simulink model "Experiment_0310yice_cs"  (R2019a)
settings: Solver=ode5  StartTime=0.0  StopTime=20  FixedStep=1/100  RelTol=1e-3
PreLoadFcn:
  | mbxruntime.callbacks.PreLoadFcn(bdroot);
PostLoadFcn:
  | mbxruntime.callbacks.PostLoadFcn(bdroot);
InitFcn:
  | mbxruntime.callbacks.InitFcn(bdroot);
StartFcn:
  | mbxruntime.callbacks.StartFcn(bdroot);
StopFcn:
  | mbxruntime.callbacks.StopFcn(bdroot);
model workspace (MAT data in the model file):
  mbox_table : struct (value not decoded)
  model_closed = 0
  sim_status = 0
undefined symbols (not defined in the file or in its folder): DiscIntNeverNeededParam, InitImageOutputDir
libraries: PreScanSimulinkLibrary x20, simulink_extras x1
(part 1 of 2)
CloseFcn:
  | mbxruntime.callbacks.CloseFcn(bdroot);
settings Model: NumberOfSteps=10  Creator=PRESCAN  LastModifiedBy=HP
settings DataIOCC: LimitDataPoints=on  SaveFormat=Array  SignalLoggingSaveFormat=ModelDataLogs  ReturnWorkspaceOutputs=off
settings OptimizationCC: ExpressionDepthLimit=2147483647  InitFltsAndDblsToZero=on  LifeSpan=inf
settings DebuggingCC: SaveWithParameterizedLinksMsg=none  UnderspecifiedInitializationDetection=Classic  MergeDetectMultiDrivingBlocksExec=none  SignalResolutionControl=TryResolveAllWithWarning  MultiTaskDSMMsg=warning  MultiTaskCondExecSysMsg=none  FcnCallInpInsideContextMsg=warning  StateNameClashWarn=warning  SFUnexpectedBacktrackingDiag=warning  SFNoUnconditionalDefaultTransitionDiag=warning  SFExecutionAtInitializationDiag=none  ArithmeticOperatorsInVariantConditions=warning
settings HardwareCC: ProdBitPerPointer=32  ProdBitPerSizeT=32  ProdBitPerPtrDiffT=32  ProdLargestAtomicFloat=None  ProdIntDivRoundTo=Undefined  ProdEndianess=Unspecified  ProdWordSize=32  ProdHWDeviceType=32-bit Generic
settings ModelReferenceCC: UpdateModelReferenceTargets=IfOutOfDate  PropagateSignalLabelsOutOfModel=off
settings SFSimCC: SimUseLocalCustomCode=off  SimParseCustomCode=off
settings SFSimCC: SimCustomHeaderCode=|
  | #include "prescan.h"
  | #include "prescan_platform.h"
settings RTWCC: RTWUseLocalCustomCode=off
settings CodeAppCC: StateflowObjectComments=on
settings GRTTargetCC: TargetFcnLib=ansi_tfl_tmw.mat  TargetLangStandard=C89/C90 (ANSI)  GeneratePreprocessorConditionals=Disable all  CombineOutputUpdateFcns=off  GRTInterface=on
settings ConfigComp: CovMetricSettings=dw  CovHtmlReporting=on  CovSaveCumulativeToWorkspaceVar=on  CovSaveSingleToWorkspaceVar=on  CovExternalEMLEnable=off

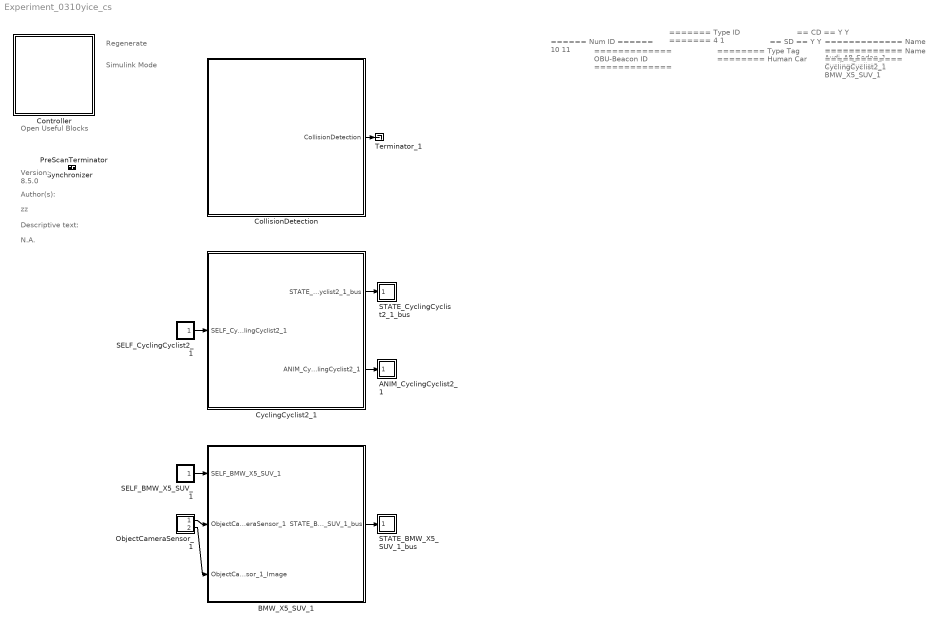
== system Experiment_0310yice_cs ==
  note: Regenerate
  note: Simulink Mode
  note: Open Useful Blocks
  note: 8.5.0
  note: Version:
  note: Author(s):
  note: zz
  note: Descriptive text:
  note: N.A.
  note: =============
      | Name
      | =============
      | Audi_A8_Sedan_1
      | CyclingCyclist2_1
  note: ======
      | Num ID
      | ======
      | 10
      | 11
  note: =============
      | OBU-Beacon ID
      | =============
  note: =======
      | Type ID
      | =======
      | 4
      | 1
  note: ========
      | Type Tag
      | ========
      | Human
      | Car
  note: ==
      | SD
      | ==
      | Y
      | Y
  note: ==
      | CD
      | ==
      | Y
      | Y
  note: =============
      | Name
      | =============
      | CyclingCyclist2_1
      | BMW_X5_SUV_1
  ANIM_CyclingCyclist2_1 : Subsystem  Tag=actuator/AnimationOutport  Priority=0  LoadFcn=load('PreScanAnimActuatorData.mat')  mask(PreScan Sink Block: State Animation){}
      mask help: The Cyclist Animation port allows the cyclist to ride the bicycle.
      settings: OpenFcn=open_system([gcb '/Actuator'],'mask')
      mask Help: eval('openHelp(239)')
      mask Display: image(imread('CyclingCyclist2.jpg'))
  BMW_X5_SUV_1 : Subsystem  Tag=WorldObjectSubSystem  InitFcn=UniqueId = '197';
      mask init:
      | modelPath = GenericModelHelper.getGenericModelFilePath('ModelDepo','Vehicles\BMW_X5\BMW_X5.pgmb','cea918691563e9ae3e6a88ec95e6726a');imagePath = GenericModelHelper.getCompilationPicture(modelPath, 'BMW_X5_HighPoly.png');
      mask Display: image(imread(imagePath));color('white');text(0, 0, ' ID=11\n')
  CollisionDetection : Subsystem  Tag=sensor/CollisionDetection  Priority=3  LoadFcn=load('PrescanCollisionDetectionData.mat');load('PrescanCollisionDetectionMessage.mat')  mask(PreScan Source Block: CollisionDetection){}
      mask help: Collision Detection can be used to detect collisions between PreScan components. For Collision Detection the actual component shape is taken into account, so it is not a bounding box approach.
      settings: OpenFcn=open_system([gcb '/Sensor'],'mask')
      mask Help: eval('openHelp(811)')
      mask Display: image(imread('crash.jpg'))
  Controller : Subsystem  Description=C9959BB6F9C6CCCA2A6EA89AF77C45A9E7A5C62A073B3FDCE97DBD876D9D5A7D  Priority=-1  LoadFcn=load PreScanControllerData  mask(PreScan Simulation Controller){prescanversion='8.5.0', ModelReferencing=off, TimeStep=5/100, ControlMode=0, PreScanExecutionMode=on, ControllerCount=0, ControllerIndex=0, ControllerOptions=''}
      mask prompts: prescanversion "PreScan Version"; ModelReferencing "Use Model Referencing"; TimeStep "Upload Period [s]"; ControlMode "Control Mode"; PreScanExecutionMode "Execution Mode"; ControllerCount "Controller Count"; ControllerIndex "Controller Index"; ControllerOptions "Controller Options"
      mask help:
      | Please do not remove this block from the compilation sheet,
      | as it connects the model to the PreScan environment.
      mask init:
      | model = bdroot(gcb);
      | ExperimentFile = mbxruntime.findExperimentFile(model,true); %relative path
      | 
      | [d1, d2, d3, prescandata] = prescan_Settings();
      | ModelDepo = fullfile(prescandata,'ModelDepo'); 
      | 
      | RTmode = mbxruntime.getRTMode(model);
      | 
      | SimulationMode = get_param(bdroot,'SimulationMode');
      | if strcmp(SimulationMode, 'rapid-accelerator')
      |     SimulationMode = 'external';
      | end
      | TargetName = get_param(bdroot,'SystemTargetFile');
      settings: ModelCloseFcn=assignin('base',['model_closed_' bdroot],true);
      mask Help: eval('openHelp(812)')
      mask Display: image(imread('prescanlogo.ico'))
  CyclingCyclist2_1 : Subsystem  Tag=WorldObjectSubSystem  InitFcn=UniqueId = '71';
      mask init:
      | imagePath=which('CyclingCyclist2.jpg');
      mask Display: image(imread(imagePath));color('white');text(0, 0, ' ID=10\n')
  ObjectCameraSensor_1 : Subsystem  Tag=sensor/ObjectCamera/data  Priority=3  LoadFcn=load('PrescanOCSData.mat');load('PrescanOCSMessage.mat')  mask(PreScan Source Block: Object Camera Sensor){}
      mask help: The Object Camera Sensor provides information on objects locations.
      settings: OpenFcn=open_system([gcb '/Sensor'],'mask')
      mask Help: eval('openHelp(2401)')
      mask Display: image(imread('ObjectCameraSensorSL.png'))
  PreScanTerminator : Subsystem  Tag=PreScanTerminator  Priority=999  LoadFcn=load PrescanTerminatorData  mask(PreScan Simulation Terminator){TimeStep=5/100}
      mask prompts: TimeStep "Upload Period [s]"
      mask help:
      | Please do not remove this block from the compilation sheet as it
      | connects the model to the PreScan environment.
      mask Help: eval('openHelp(812)')
      mask Display: image(imread('prescanlogo.ico'))
  SELF_BMW_X5_SUV_1 : Subsystem  Tag=sensor/SelfPort  Priority=3  LoadFcn=load('PreScanSelfSensorData.mat')  mask(PreScan Source Block: SELF){}
      mask help:
      | The SELF port shows (state) information of the actor itself. The outputs are position in the experiment's axis system and the GPS coordinates, and the object's absolute velocity and compass heading.
      |
      | For more information, please click Help.
      settings: OpenFcn=open_system([gcb '/Sensor'],'mask')
      mask Help: eval('openHelp(462)')
      mask Display: image(imread('GPS.png'))
  SELF_CyclingCyclist2_1 : Subsystem  Tag=sensor/SelfPort  Priority=3  LoadFcn=load('PreScanSelfSensorData.mat')  mask(PreScan Source Block: SELF){}
      mask help:
      | The SELF port shows (state) information of the actor itself. The outputs are position in the experiment's axis system and the GPS coordinates, and the object's absolute velocity and compass heading.
      |
      | For more information, please click Help.
      settings: OpenFcn=open_system([gcb '/Sensor'],'mask')
      mask Help: eval('openHelp(462)')
      mask Display: image(imread('GPS.png'))
  STATE_BMW_X5_SUV_1_bus : Subsystem  Tag=actuator/StatePort  Priority=0  LoadFcn=load('PreScanStateActuatorData.mat')  mask(PreScan Sink Block: State){}
      mask help:
      | The Actor State contains a vector signal of size (9x1), containing the following signals:
      |
      | -  Position    	(x,y,z)             	[m]
      | -  Velocity    	(vx,vy,vz)         	[m/s]
      | -  Angles       	(Roll, Pitch, Yaw)	[rad]
      |
      | The Actor state is defined in the global axis system.
      | The state is superponed on the Initial position defined in the GUI.
      |
      | For more information, please click Help.
      settings: OpenFcn=open_system([gcb '/Actuator'],'mask')
      mask Help: eval('openHelp(222)')
      mask Display: image(imread('State.png'))
  STATE_CyclingCyclist2_1_bus : Subsystem  Tag=actuator/StatePort  Priority=0  LoadFcn=load('PreScanStateActuatorData.mat')  mask(PreScan Sink Block: State){}
      mask help:
      | The Actor State contains a vector signal of size (9x1), containing the following signals:
      |
      | -  Position    	(x,y,z)             	[m]
      | -  Velocity    	(vx,vy,vz)         	[m/s]
      | -  Angles       	(Roll, Pitch, Yaw)	[rad]
      |
      | The Actor state is defined in the global axis system.
      | The state is superponed on the Initial position defined in the GUI.
      |
      | For more information, please click Help.
      settings: OpenFcn=open_system([gcb '/Actuator'],'mask')
      mask Help: eval('openHelp(222)')
      mask Display: image(imread('State.png'))
  Synchronizer : Subsystem  Tag=PreScanSynchronizer  Priority=1  LoadFcn=load PrescanSynchronizeData  mask(PreScan Simulation Core Block){TimeStep=5/100}
      mask prompts: TimeStep "Timestep [s]"
      mask help:
      | Please do not remove this block from the PreScan compilation sheet,
      | as it contains essential configuration parameters for a PreScan simulation.
      settings: DeleteFcn=PreScanBlockDeleteFcn;
      mask Display: image(imread('prescanlogo.ico'))
  Terminator_1 : Terminator
  wires:
  CyclingCyclist2_1/1(STATE_CyclingCyclist2_1_bus) -> STATE_CyclingCyclist2_1_bus/1(STATE_CyclingCyclist2_1_bus)
  CyclingCyclist2_1/2(ANIM_CyclingCyclist2_1) -> ANIM_CyclingCyclist2_1/1(ANIM_CyclingCyclist2_1)
  SELF_CyclingCyclist2_1/1(SELF_CyclingCyclist2_1) -> CyclingCyclist2_1/1(SELF_CyclingCyclist2_1)
  CollisionDetection/1(CollisionDetection) -> Terminator_1/1
  BMW_X5_SUV_1/1(STATE_BMW_X5_SUV_1_bus) -> STATE_BMW_X5_SUV_1_bus/1(STATE_BMW_X5_SUV_1_bus)
  SELF_BMW_X5_SUV_1/1(SELF_BMW_X5_SUV_1) -> BMW_X5_SUV_1/1(SELF_BMW_X5_SUV_1)
  ObjectCameraSensor_1/1(ObjectCameraSensor_1) -> BMW_X5_SUV_1/2(ObjectCameraSensor_1)
  ObjectCameraSensor_1/2(ObjectCameraSensor_1_Image) -> BMW_X5_SUV_1/3(ObjectCameraSensor_1_Image)

== system Experiment_0310yice_cs/ANIM_CyclingCyclist2_1 ==
  ANIM_CyclingCyclist2_1 : Inport  Tag=inport/AnimationOutport  OutDataTypeStr=Bus: PRESCAN_ANIMACTUATORDATA  PortDimensions=2  SampleTime=5/100  BusOutputAsStruct=on
  Actuator : S-Function  FunctionName=sfun_CyclistAnimActuator  Parameters=UniqueID, uint8([ParentObject 0]), TimeStep  SFunctionDeploymentMode=off  EnableBusSupport=off  mask(PreScan Sink Block: State Animation){UniqueID=71, ParentObject=CyclingCyclist2_1, TimeStep=5/100}
      mask prompts: UniqueID "Auto-Assigned: Unique ID"; ParentObject "Auto-Assigned: ParentObject"; TimeStep "Auto-Assigned: Upload Period [s]"
      mask help: The Cyclist Animation port allows the cyclist to ride the bicycle.
      mask Help: eval('openHelp(239)')
      mask Display: image(imread('CyclingCyclist2.jpg'))
  wires:
  ANIM_CyclingCyclist2_1/1 -> Actuator/1

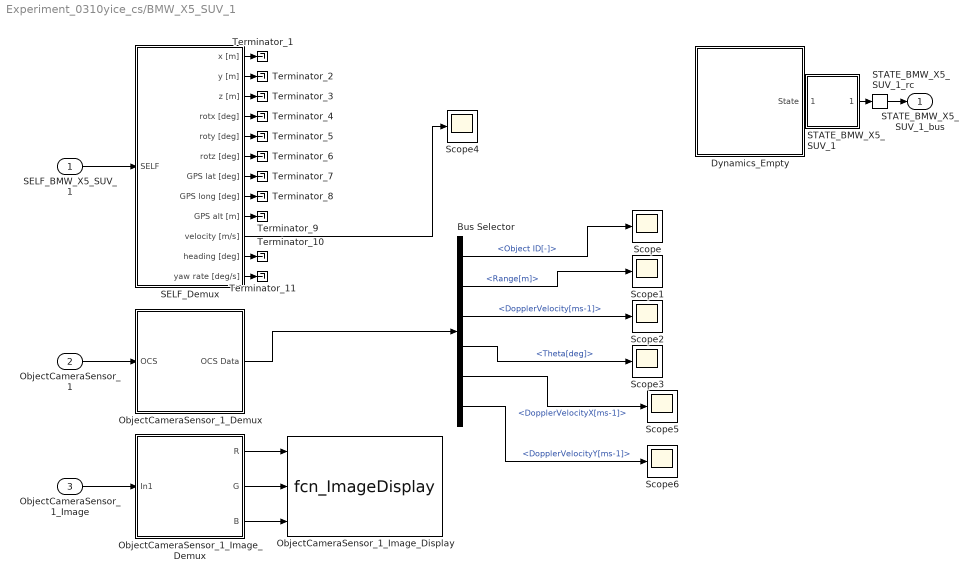
== system Experiment_0310yice_cs/BMW_X5_SUV_1 ==
  SELF_BMW_X5_SUV_1 : Inport  Tag=inport/SelfPort  OutDataTypeStr=Bus: PRESCAN_SELFSENSORDATA  PortDimensions=1  SampleTime=5/100  BusOutputAsStruct=on
  ObjectCameraSensor_1 : Inport  Tag=inport/ObjectCamera/data  Port=2  OutDataTypeStr=Bus: PRESCAN_OCS_MESSAGE  PortDimensions=3  SampleTime=1/20  BusOutputAsStruct=on
  ObjectCameraSensor_1_Image : Inport  Tag=inport/ObjectCamera/image  Port=3  OutDataTypeStr=uint8  SampleTime=1/20  BusOutputAsStruct=on
  Bus Selector : BusSelector  OutputSignals=Object ID[-],Range[m],DopplerVelocity[ms-1],Theta[deg],DopplerVelocityX[ms-1],DopplerVelocityY[ms-1]
  Dynamics_Empty : Subsystem  Tag=Dynamics_Empty
      mask Help: eval('openHelp(202)')
      mask Display: port_label('output', 1, 'State');text(0,0,' Empty\n')
  ObjectCameraSensor_1_Demux : Subsystem  Tag=demux/OCS  mask(PreScan Demux Block: Object Camera Sensor){detectableObjects=3}
      mask prompts: detectableObjects "Max. detectable objects"
      settings: DeleteFcn=PreScanBlockDeleteFcn;
      mask Help: eval('openHelp(2401)')
      mask Display:
      | port_label('input', 1, 'OCS')
      | port_label('output', 1, 'OCS Data')
  ObjectCameraSensor_1_Image_Demux : Subsystem  Tag=demux/Camera/Color  mask{SensorName=ObjectCameraSensor_1, hres=320, vres=240}
      mask prompts: SensorName "Sensor Name"; hres "Horizontal Resolution"; vres "Vertical Resolution"
      mask Help: eval('openHelp(2401)')
      mask Display:
      | fprintf('MONO CAMERA:\n Color\n %s \n %d x %d px',SensorName,hres,vres)
      | port_label('output',1,'R')
      | port_label('output',2,'G')
      | port_label('output',3,'B')
  ObjectCameraSensor_1_Image_Display : M-S-Function  Tag=CameraSensor_Color_Display  InitFcn=InitImageOutputDir(gcb);  FunctionName=fcn_ImageDisplay  Parameters=SensorName EnableDisplay EnablePosition DisplayPosition FigureHandle SaveResults BitmapFormat TempOutputDir CameraType DataType  mask(PreScan Color Display Block){SensorName=ObjectCameraSensor_1_Image, EnableDisplay=on, EnablePosition=off, DisplayPosition=[10 10 320 240], FigureHandle=19701, SaveResults=off, Format=PNG, TempOutputDir=0, CameraType=Mono, DataType=uint8}
      mask prompts: SensorName "User Specified: Title of Display"; EnableDisplay "Active"; EnablePosition "Set Display window position"; DisplayPosition "Display window position [xpos ypos width height]"; FigureHandle "Unique Handle"; SaveResults "Save results"; TempOutputDir "OutputDir"; CameraType "Camera Type"; DataType "Image Data Type"
      mask help: This block displays the RGB output of a PreScan camera sensor.
      mask init:
      | if EnableDisplay
      |     EnableString='';
      |     EnableColor='gray';
      | else
      |     EnableString='INACTIVE';
      |     EnableColor='red';
      | end
      | switch Format
      |     case 1
      |         BitmapFormat = 'png';
      |     case 2
      |         BitmapFormat = 'bmp';
      |     case 3
      |         BitmapFormat = 'jpg';
      | end 
      | if CameraType==1
      |     CameraTypeName='MONO';
      |     PortNumber=0;
      | else
      |     CameraTypeName='STEREO';
      |     PortNumber=3;
      | end
      settings: CopyFcn=CopyFcnDisplay  DeleteFcn=PreScanBlockDeleteFcn;  ModelCloseFcn=fcn_ImageDisplay_ModelCloseFcn
      mask Help: eval('openHelp(2401)')
      mask Callback EnablePosition:
      | MV=get_param(gcb,'MaskVisibilities');
      | if strcmp(get_param(gcb,'EnablePosition'),'on')
      |     MV{4}='on';
      | else
      |     MV{4}='off';
      | end
      | set_param(gcb,'MaskVisibilities',MV);
      | clear MV;
      mask TypeOptions Format: PNG | BMP | JPG
      mask TypeOptions CameraType: Mono | Stereo
      mask TypeOptions DataType: uint8 | single
      mask Display:
      | color(EnableColor);
      | fprintf('%s\n DISPLAY:\n Color \n %s',EnableString,SensorName)
      | port_label('input',1,'R')
      | port_label('input',2,'G')
      | port_label('input',3,'B')
      | port_label('input',PortNumber+1,'R')
      | port_label('input',PortNumber+2,'G')
      | port_label('input',PortNumber+3,'B')
  SELF_Demux : Subsystem  Tag=demux/SelfPort  mask(PreScan Demux Block:){}
      mask help:
      | The SELF port shows (state) information of the actor itself. The outputs are position in the experiment's axis system and the GPS coordinates, and the object's absolute velocity and compass heading.
      |
      | For more information, please click Help.
      settings: DeleteFcn=PreScanBlockDeleteFcn;
      mask Help: eval('openHelp(462)')
      mask Display:
      | port_label('output',1,'x [m]')
      | port_label('output',2,'y [m]')
      | port_label('output',3,'z [m]','texmode','on')
      | port_label('output',4,'Rotx [deg]','texmode','on')
      | port_label('output',5,'Roty [deg]','texmode','on')
      | port_label('output',6,'Rotz [deg]','texmode','on')
      | port_label('output',7,'GPS lat [deg]','texmode','on')
      | port_label('output',8,'GPS long [deg]','texmode','on')
      | port_label('output',9,'GPS alt [m]','texmode','on')
      | port_label('output',10,'Velocity [m/s]')
      | port_label('output',11,'Heading [deg]')
      | port_label('output',12,'Yaw rate [deg/s]')
  STATE_BMW_X5_SUV_1 : Subsystem  Tag=mux/StatePort  Priority=0  LoadFcn=load PrescanStateActuatorData  mask(PreScan Sink Block: State){x0=44.6973, y0=48.6545, z0=0.69, Roll0=0, Pitch0=0, Yaw0=90, TimeStep=1/100}
      mask prompts: x0 "Ini x-position VEHICLE wrt GLOBAL axis system [m]"; y0 "Ini y-position VEHICLE wrt GLOBAL axis system [m]"; z0 "Ini z-position VEHICLE wrt GLOBAL axis system [m]"; Roll0 "Ini roll-angle BODY wrt VEHICLE axis system [deg]"; Pitch0 "Ini pitch-angle BODY wrt VEHICLE axis system [deg]"; Yaw0 "Ini yaw-angle VEHICLE wrt GLOBAL axis system [deg]"; TimeStep "Auto-Assigned: Upload Period [s]"
      mask help:
      | The Actor State contains a vector signal of size (9x1), containing the following signals:
      |
      | -  Position                  (x,y,z)                                     [m]
      | -  Velocity                  (vx,vy,vz)                               [m/s]
      | -  Angles                    (Roll, Pitch, Yaw)                   [rad]
      |
      | The Actor state is defined in the global axis system.
      | The state is superponed on the Initial position defined in the GUI.
      |
      | For more information, please click Help.
      settings: DeleteFcn=PreScanBlockDeleteFcn;
      mask Help: eval('openHelp(222)')
      mask Display: image(imread('State.png'))
  STATE_BMW_X5_SUV_1_rc : RateTransition  Tag=mux_rc/StatePort  OutPortSampleTimeOpt=Inherit
  Scope{,1..6} (7 alike) : Scope
  Terminator_{1..11} (11 alike) : Terminator
  STATE_BMW_X5_SUV_1_bus : Outport  Tag=outport/StatePort  OutDataTypeStr=Bus: PRESCAN_STATEACTUATORDATA  PortDimensions=1  SampleTime=5/100
  wires:
  ObjectCameraSensor_1_Demux/1(OCS Data) -> Bus Selector/1
  Bus Selector/1 -> Scope/1  "<Object ID[-]>"
  Bus Selector/2 -> Scope1/1  "<Range[m]>"
  Bus Selector/3 -> Scope2/1  "<DopplerVelocity[ms-1]>"
  Bus Selector/4 -> Scope3/1  "<Theta[deg]>"
  SELF_Demux/10(velocity [m/s]) -> Scope4/1
  Bus Selector/5 -> Scope5/1  "<DopplerVelocityX[ms-1]>"
  Bus Selector/6 -> Scope6/1  "<DopplerVelocityY[ms-1]>"
  STATE_BMW_X5_SUV_1_rc/1 -> STATE_BMW_X5_SUV_1_bus/1
  STATE_BMW_X5_SUV_1/1(StateBus) -> STATE_BMW_X5_SUV_1_rc/1
  SELF_BMW_X5_SUV_1/1 -> SELF_Demux/1(SELF)
  ObjectCameraSensor_1/1 -> ObjectCameraSensor_1_Demux/1(OCS)
  ObjectCameraSensor_1_Image/1 -> ObjectCameraSensor_1_Image_Demux/1(In1)
  ObjectCameraSensor_1_Image_Demux/1(R) -> ObjectCameraSensor_1_Image_Display/1
  ObjectCameraSensor_1_Image_Demux/2(G) -> ObjectCameraSensor_1_Image_Display/2
  ObjectCameraSensor_1_Image_Demux/3(B) -> ObjectCameraSensor_1_Image_Display/3
  Dynamics_Empty/1(State) -> STATE_BMW_X5_SUV_1/1(State)
  SELF_Demux/1(x [m]) -> Terminator_1/1
  SELF_Demux/2(y [m]) -> Terminator_2/1
  SELF_Demux/3(z [m]) -> Terminator_3/1
  SELF_Demux/4(rotx [deg]) -> Terminator_4/1
  SELF_Demux/5(roty [deg]) -> Terminator_5/1
  SELF_Demux/6(rotz [deg]) -> Terminator_6/1
  SELF_Demux/7(GPS lat [deg]) -> Terminator_7/1
  SELF_Demux/8(GPS long [deg]) -> Terminator_8/1
  SELF_Demux/9(GPS alt [m]) -> Terminator_9/1
  SELF_Demux/11(heading [deg]) -> Terminator_10/1
  SELF_Demux/12(yaw rate [deg/s]) -> Terminator_11/1

== system Experiment_0310yice_cs/CollisionDetection ==
  Sensor : S-Function  FunctionName=sfun_CollisionDetection  Parameters=detectableCollisions, timestep  SFunctionDeploymentMode=off  EnableBusSupport=off  mask(PreScan Source Block: CollisionDetection){detectableCollisions=5, timestep=5/100}
      mask prompts: detectableCollisions "Max detectable collisions:"; timestep "MATLAB timestep:"
      mask help: Collision Detection can be used to detect collisions between PreScan components. For Collision Detection the actual component shape is taken into account, so it is not a bounding box approach.
      mask Help: eval('openHelp(811)')
      mask Display: image(imread('crash.jpg'))
  CollisionDetection : Outport  Tag=outport/CollisionDetection  OutDataTypeStr=Bus: PRESCAN_COLLISIONDETECTION_MESSAGE  PortDimensions=5  SampleTime=5/100
  wires:
  Sensor/1 -> CollisionDetection/1

== system Experiment_0310yice_cs/Controller ==
  Terminator : Terminator
  sfun_Controller : S-Function  FunctionName=sfun_Controller  Parameters=SParameter1, SParameter2, SParameter3, SParameter4, SParameter5, SParameter6, SParameter7, SParameter8, SParameter9, SParameter10, SampleTime  SFunctionDeploymentMode=off  EnableBusSupport=off  mask(Legacy Function){SFunctionSpec=void prescan_outputFcn(void** work1, PRESCAN_CONTROLLERDATA y1[1]), SParameter1=uint8([ExperimentFile 0]), SParameter2=uint8([ModelDepo 0]), SParameter3=uint8([ControllerOptions 0]), SParameter4=RTmode, SParameter5=PreScanExecutionMode, SParameter6=ControlMode, SParameter7=ControllerCount, SParameter8=ControllerIndex, SParameter9=uint8([SimulationMode 0]), SParameter10=uint8([TargetName 0]), SampleTime=TimeStep, ShowSpec=on}
      mask prompts: SParameter1 "P1:"; SParameter2 "P2:"; SParameter3 "P3:"; SParameter4 "P4:"; SParameter5 "P5:"; SParameter6 "P6:"; SParameter7 "P7:"; SParameter8 "P8:"; SParameter9 "P9:"; SParameter10 "P10:"; SampleTime "Sample time (-1 for inherited):"; ShowSpec "Display function specification"
      mask help:
      | This block allows you to call the legacy functions specified by the following Legacy Code Tool definition:
      | def.SFunctionName = 'sfun_Controller';
      | def.OutputFcnSpec = 'void prescan_outputFcn(void** work1, PRESCAN_CONTROLLERDATA y1[1])';
      | def.StartFcnSpec = 'void prescan_startFcn(void ** work1, uint8 p1[], uint8 p2[], uint8 p3[], double p4, double p5, double p6, double p7, double p8, uint8 p9[], uint8 p10[])';
      | def.TerminateFcnSpec = 'void prescan_terminateFcn(void** work1)';
      | def.HeaderFiles = {'prescan_controller_data.h', 'prescan_SFunLibrary.h', 'prescan_CreateLogHandler.h', 'prescan_CreateErrorHandler.h', 'prescan_modify.h', 'ModuleDLL.h'};
      | def.SourceFiles = {'prescan_MexLogHandler.c', 'prescan_SimStructErrorHandler.c', 'prescan_LogHandler.c', 'prescan_ErrorHandler.c', 'prescan_Modify.c'};
      | def.HostLibFiles = {'sensorinterfaced.lib'};
      | def.TargetLibFiles = {'sensorinterfaced.so'};
      | def.IncPaths = {'.', 'C:\projects\prescan\rt_vislibrary\vis\..\pimp\include\sensors\InterfaceRTW'};
      | def.SrcPaths = {'C:\projects\prescan\rt_vislibrary\vis\..\pimp\include\sensors\InterfaceRTW', 'C:\projects\prescan\rt_vislibrary\vis\..\pimp\include\sensors\InterfaceRTW\ccurrt'};
      | def.LibPaths = {'C:\\projects\\prescan\\vislibrary_build\lib'};
      | def.SampleTime = 'parameterized';
      mask Help: <p>This block was generated automatically by the Legacy Code Tool. For detailed help on this tool, call<a href="matlab:legacy_code('help')"> legacy_code('help')</a>.</p>
      mask Callback ShowSpec:
      | if strcmp(get_param(gcbh, 'ShowSpec'), 'on')
      |   set_param(gcbh, 'MaskDisplay', sprintf('fprintf(''%s'');', get_param(gcbh, 'SFunctionSpec')));
      | else
      |   set_param(gcbh, 'MaskDisplay', sprintf('fprintf(''%s'');', get_param(gcbh, 'FunctionName')));
      | end
      mask Display: fprintf('void prescan_outputFcn(void** work1, PRESCAN_CONTROLLERDATA y1[1])');
  wires:
  sfun_Controller/1 -> Terminator/1

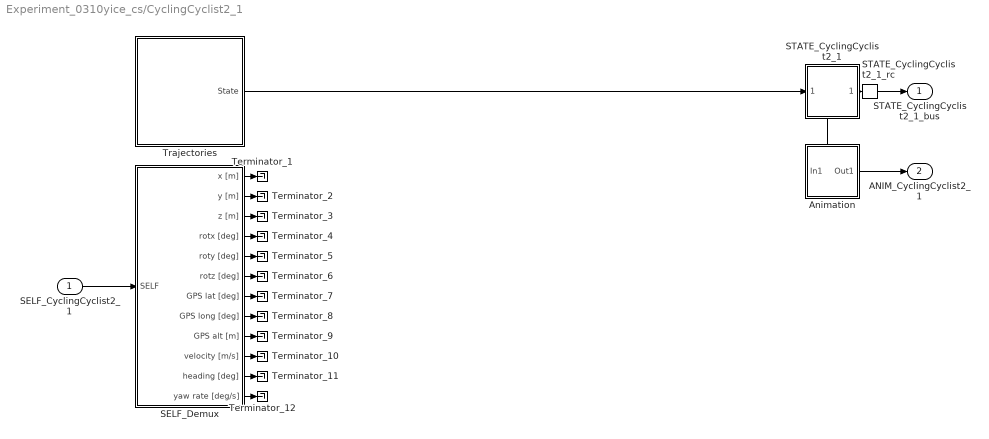
== system Experiment_0310yice_cs/CyclingCyclist2_1 ==
  SELF_CyclingCyclist2_1 : Inport  Tag=inport/SelfPort  OutDataTypeStr=Bus: PRESCAN_SELFSENSORDATA  PortDimensions=1  SampleTime=5/100  BusOutputAsStruct=on
  Animation : Subsystem  Tag=CyclistAnimation  mask(Prescan Conversion Block: Cyclist Animation){TimeStep=5/100}
      mask prompts: TimeStep "Auto-Assigned: Upload Period [s]"
      mask help: The Cyclist animation block converts the State signal into the animation signal for proper animation of the cycling cyclist.
      mask Help: eval('openHelp(239)');
      mask Display: image(imread('CyclingCyclist2.jpg'));
  SELF_Demux : Subsystem  Tag=demux/SelfPort  mask(PreScan Demux Block:){}
      mask help:
      | The SELF port shows (state) information of the actor itself. The outputs are position in the experiment's axis system and the GPS coordinates, and the object's absolute velocity and compass heading.
      |
      | For more information, please click Help.
      settings: DeleteFcn=PreScanBlockDeleteFcn;
      mask Help: eval('openHelp(462)')
      mask Display:
      | port_label('output',1,'x [m]')
      | port_label('output',2,'y [m]')
      | port_label('output',3,'z [m]','texmode','on')
      | port_label('output',4,'Rotx [deg]','texmode','on')
      | port_label('output',5,'Roty [deg]','texmode','on')
      | port_label('output',6,'Rotz [deg]','texmode','on')
      | port_label('output',7,'GPS lat [deg]','texmode','on')
      | port_label('output',8,'GPS long [deg]','texmode','on')
      | port_label('output',9,'GPS alt [m]','texmode','on')
      | port_label('output',10,'Velocity [m/s]')
      | port_label('output',11,'Heading [deg]')
      | port_label('output',12,'Yaw rate [deg/s]')
  STATE_CyclingCyclist2_1 : Subsystem  Tag=mux/StatePort  Priority=0  LoadFcn=load PrescanStateActuatorData  mask(PreScan Sink Block: State){x0=34.5734, y0=102.2433, z0=0, Roll0=0, Pitch0=0, Yaw0=270, TimeStep=5/100}
      mask prompts: x0 "Ini x-position VEHICLE wrt GLOBAL axis system [m]"; y0 "Ini y-position VEHICLE wrt GLOBAL axis system [m]"; z0 "Ini z-position VEHICLE wrt GLOBAL axis system [m]"; Roll0 "Ini roll-angle BODY wrt VEHICLE axis system [deg]"; Pitch0 "Ini pitch-angle BODY wrt VEHICLE axis system [deg]"; Yaw0 "Ini yaw-angle VEHICLE wrt GLOBAL axis system [deg]"; TimeStep "Auto-Assigned: Upload Period [s]"
      mask help:
      | The Actor State contains a vector signal of size (9x1), containing the following signals:
      |
      | -  Position                  (x,y,z)                                     [m]
      | -  Velocity                  (vx,vy,vz)                               [m/s]
      | -  Angles                    (Roll, Pitch, Yaw)                   [rad]
      |
      | The Actor state is defined in the global axis system.
      | The state is superponed on the Initial position defined in the GUI.
      |
      | For more information, please click Help.
      settings: DeleteFcn=PreScanBlockDeleteFcn;
      mask Help: eval('openHelp(222)')
      mask Display: image(imread('State.png'))
  STATE_CyclingCyclist2_1_rc : RateTransition  Tag=mux_rc/StatePort  OutPortSampleTimeOpt=Inherit
  Terminator_{1..12} (12 alike) : Terminator
  Trajectories : Subsystem  Tag=Trajectories  mask(PreScan Source Block: Trajectories){}
      mask help:
      | The Trajectory block contains the trajectories defined in the PreScan Experiment Editor. The output of the trajectory block is the (vehicle) State.
      |
      | For more information, please click Help.
      settings: DeleteFcn=PreScanBlockDeleteFcn;
      mask Help: eval('openHelp(312)')
      mask Display: image(imread('Trajectory.png'));
  STATE_CyclingCyclist2_1_bus : Outport  Tag=outport/StatePort  OutDataTypeStr=Bus: PRESCAN_STATEACTUATORDATA  PortDimensions=1  SampleTime=5/100
  ANIM_CyclingCyclist2_1 : Outport  Tag=outport/AnimationOutport  Port=2  OutDataTypeStr=Bus: PRESCAN_ANIMACTUATORDATA  PortDimensions=2  SampleTime=5/100
  wires:
  STATE_CyclingCyclist2_1_rc/1 -> STATE_CyclingCyclist2_1_bus/1
  STATE_CyclingCyclist2_1/1(StateBus) -> STATE_CyclingCyclist2_1_rc/1, Animation/1(In1)
  Animation/1(Out1) -> ANIM_CyclingCyclist2_1/1
  SELF_CyclingCyclist2_1/1 -> SELF_Demux/1(SELF)
  Trajectories/1(State) -> STATE_CyclingCyclist2_1/1(State)
  SELF_Demux/1(x [m]) -> Terminator_1/1
  SELF_Demux/2(y [m]) -> Terminator_2/1
  SELF_Demux/3(z [m]) -> Terminator_3/1
  SELF_Demux/4(rotx [deg]) -> Terminator_4/1
  SELF_Demux/5(roty [deg]) -> Terminator_5/1
  SELF_Demux/6(rotz [deg]) -> Terminator_6/1
  SELF_Demux/7(GPS lat [deg]) -> Terminator_7/1
  SELF_Demux/8(GPS long [deg]) -> Terminator_8/1
  SELF_Demux/9(GPS alt [m]) -> Terminator_9/1
  SELF_Demux/10(velocity [m/s]) -> Terminator_10/1
  SELF_Demux/11(heading [deg]) -> Terminator_11/1
  SELF_Demux/12(yaw rate [deg/s]) -> Terminator_12/1

== system Experiment_0310yice_cs/ObjectCameraSensor_1 ==
  Sensor : S-Function  FunctionName=sfun_OCS  Parameters=sensorID, detectableObjects, dataWidth, dataHeight, channelsPerImage, timestep  SFunctionDeploymentMode=off  EnableBusSupport=off  mask(PreScan Source Block: Object Camera Sensor){sensorID=198, detectableObjects=3, dataWidth=240, dataHeight=960, channelsPerImage=3, timestep=1/20}
      mask prompts: sensorID "Sensor ID"; detectableObjects "Max detectable objects:"; dataWidth "Data width"; dataHeight "Data Height"; channelsPerImage "Channels per image"; timestep "MATLAB timestep:"
      mask help: The Object Camera Sensor provides information on objects locations.
      mask Help: eval('openHelp(2401)')
      mask Display: image(imread('ObjectCameraSensorSL.png'))
  ObjectCameraSensor_1 : Outport  Tag=outport/ObjectCamera/data  OutDataTypeStr=Bus: PRESCAN_OCS_MESSAGE  PortDimensions=3  SampleTime=1/20
  ObjectCameraSensor_1_Image : Outport  Tag=outport/ObjectCamera/image  Port=2  OutDataTypeStr=uint8  SampleTime=1/20
  wires:
  Sensor/1 -> ObjectCameraSensor_1/1
  Sensor/2 -> ObjectCameraSensor_1_Image/1

== system Experiment_0310yice_cs/PreScanTerminator ==
  Terminator : Terminator
  sfun_Terminator : S-Function  FunctionName=sfun_Terminator  Parameters=SampleTime  SFunctionDeploymentMode=off  EnableBusSupport=off  mask(Legacy Function){SFunctionSpec=void prescan_terminator_outputFcn(void ** work1, PRESCAN_TERMINATORDATA y1[1]), SampleTime=TimeStep, ShowSpec=on}
      mask prompts: SampleTime "Sample time (-1 for inherited):"; ShowSpec "Display function specification"
      mask help:
      | This block allows you to call the legacy functions specified by the following Legacy Code Tool definition:
      | def.SFunctionName = 'sfun_Terminator';
      | def.OutputFcnSpec = 'void prescan_terminator_outputFcn(void ** work1, PRESCAN_TERMINATORDATA y1[1])';
      | def.StartFcnSpec = 'void prescan_terminator_startFcn(void ** work1)';
      | def.TerminateFcnSpec = 'void prescan_terminator_terminateFcn(void ** work1)';
      | def.HeaderFiles = {'prescan_terminator_data.h'};
      | def.HostLibFiles = {'sensorinterfaced.lib'};
      | def.IncPaths = {'src', 'C:\prescandev\vislibrary\vis\..\pimp\include\sensors\InterfaceRTW'};
      | def.SrcPaths = {'src'};
      | def.LibPaths = {'C:\\prescandev\\vislibrary_build\lib'};
      | def.SampleTime = 'parameterized';
      | def.Options.language = 'C';
      mask Help: <p>This block was generated automatically by the Legacy Code Tool. For detailed help on this tool, call<a href="matlab:legacy_code('help')"> legacy_code('help')</a>.</p>
      mask Callback ShowSpec:
      | if strcmp(get_param(gcbh, 'ShowSpec'), 'on')
      |   set_param(gcbh, 'MaskDisplay', sprintf('fprintf(''%s'');', get_param(gcbh, 'SFunctionSpec')));
      | else
      |   set_param(gcbh, 'MaskDisplay', sprintf('fprintf(''%s'');', get_param(gcbh, 'FunctionName')));
      | end
      mask Display: fprintf('void prescan_terminator_outputFcn(void ** work1, PRESCAN_TERMINATORDATA y1[1])');
  wires:
  sfun_Terminator/1 -> Terminator/1

== system Experiment_0310yice_cs/SELF_BMW_X5_SUV_1 ==
  Sensor : S-Function  FunctionName=sfun_SelfSensor  Parameters=UniqueID, TimeStep  SFunctionDeploymentMode=off  EnableBusSupport=off  mask(PreScan Source Block: SELF){UniqueID=197, TimeStep=5/100}
      mask prompts: UniqueID "Auto-Assigned: Unique ID"; TimeStep "Auto-Assigned: Upload Period [s]"
      mask help:
      | The SELF port shows (state) information of the actor itself. The outputs are position in the experiment's axis system and the GPS coordinates, and the object's absolute velocity and compass heading.
      |
      | For more information, please click Help.
      mask Help: eval('openHelp(462)')
      mask Display: image(imread('GPS.png'))
  SELF_BMW_X5_SUV_1 : Outport  Tag=outport/SelfPort  OutDataTypeStr=Bus: PRESCAN_SELFSENSORDATA  PortDimensions=1  SampleTime=5/100
  wires:
  Sensor/1 -> SELF_BMW_X5_SUV_1/1

== system Experiment_0310yice_cs/SELF_CyclingCyclist2_1 ==
  Sensor : S-Function  FunctionName=sfun_SelfSensor  Parameters=UniqueID, TimeStep  SFunctionDeploymentMode=off  EnableBusSupport=off  mask(PreScan Source Block: SELF){UniqueID=71, TimeStep=5/100}
      mask prompts: UniqueID "Auto-Assigned: Unique ID"; TimeStep "Auto-Assigned: Upload Period [s]"
      mask help:
      | The SELF port shows (state) information of the actor itself. The outputs are position in the experiment's axis system and the GPS coordinates, and the object's absolute velocity and compass heading.
      |
      | For more information, please click Help.
      mask Help: eval('openHelp(462)')
      mask Display: image(imread('GPS.png'))
  SELF_CyclingCyclist2_1 : Outport  Tag=outport/SelfPort  OutDataTypeStr=Bus: PRESCAN_SELFSENSORDATA  PortDimensions=1  SampleTime=5/100
  wires:
  Sensor/1 -> SELF_CyclingCyclist2_1/1

== system Experiment_0310yice_cs/STATE_BMW_X5_SUV_1_bus ==
  STATE_BMW_X5_SUV_1_bus : Inport  Tag=inport/StatePort  OutDataTypeStr=Bus: PRESCAN_STATEACTUATORDATA  PortDimensions=1  SampleTime=5/100  BusOutputAsStruct=on
  Actuator : S-Function  FunctionName=sfun_StateActuator  Parameters=UniqueID, TimeStep  SFunctionDeploymentMode=off  EnableBusSupport=off  mask(PreScan Sink Block: State){UniqueID=197, TimeStep=5/100}
      mask prompts: UniqueID "Auto-Assigned: Unique ID"; TimeStep "Auto-Assigned: Upload Period [s]"
      mask help:
      | The Actor State contains a vector signal of size (9x1), containing the following signals:
      |
      | -  Position    	(x,y,z)             	[m]
      | -  Velocity    	(vx,vy,vz)         	[m/s]
      | -  Angles       	(Roll, Pitch, Yaw)	[rad]
      |
      | The Actor state is defined in the global axis system.
      | The state is superponed on the Initial position defined in the GUI.
      |
      | For more information, please click Help.
      mask Help: eval('openHelp(222)')
      mask Display: image(imread('State.png'))
  wires:
  STATE_BMW_X5_SUV_1_bus/1 -> Actuator/1

== system Experiment_0310yice_cs/STATE_CyclingCyclist2_1_bus ==
  STATE_CyclingCyclist2_1_bus : Inport  Tag=inport/StatePort  OutDataTypeStr=Bus: PRESCAN_STATEACTUATORDATA  PortDimensions=1  SampleTime=5/100  BusOutputAsStruct=on
  Actuator : S-Function  FunctionName=sfun_StateActuator  Parameters=UniqueID, TimeStep  SFunctionDeploymentMode=off  EnableBusSupport=off  mask(PreScan Sink Block: State){UniqueID=71, TimeStep=5/100}
      mask prompts: UniqueID "Auto-Assigned: Unique ID"; TimeStep "Auto-Assigned: Upload Period [s]"
      mask help:
      | The Actor State contains a vector signal of size (9x1), containing the following signals:
      |
      | -  Position    	(x,y,z)             	[m]
      | -  Velocity    	(vx,vy,vz)         	[m/s]
      | -  Angles       	(Roll, Pitch, Yaw)	[rad]
      |
      | The Actor state is defined in the global axis system.
      | The state is superponed on the Initial position defined in the GUI.
      |
      | For more information, please click Help.
      mask Help: eval('openHelp(222)')
      mask Display: image(imread('State.png'))
  wires:
  STATE_CyclingCyclist2_1_bus/1 -> Actuator/1

== system Experiment_0310yice_cs/Synchronizer ==
  Bus Selector1 : BusSelector  OutputSignals=FederateStopped
  Stop Simulation : Stop
  sfun_Synchronizer : S-Function  FunctionName=sfun_Synchronizer  Parameters=SampleTime  SFunctionDeploymentMode=off  EnableBusSupport=off  mask(Legacy Function){SFunctionSpec=void prescan_synchronizer_outputFcn(void ** work1, PRESCAN_SYNCHRONIZEDATA y1[1]), SampleTime=TimeStep, ShowSpec=on}
      mask prompts: SampleTime "Sample time (-1 for inherited):"; ShowSpec "Display function specification"
      mask help:
      | This block allows you to call the legacy functions specified by the following Legacy Code Tool definition:
      | def.SFunctionName = 'sfun_Synchronizer';
      | def.OutputFcnSpec = 'void prescan_synchronizer_outputFcn(void ** work1, PRESCAN_SYNCHRONIZEDATA y1[1])';
      | def.StartFcnSpec = 'void prescan_synchronizer_startFcn(void ** work1)';
      | def.TerminateFcnSpec = 'void prescan_synchronizer_terminateFcn(void ** work1)';
      | def.HeaderFiles = {'prescan_synchronizer_data.h'};
      | def.HostLibFiles = {'sensorinterfaced.lib'};
      | def.IncPaths = {'src', 'C:\prescandev\vislibrary\vis\..\pimp\include\sensors\InterfaceRTW'};
      | def.SrcPaths = {'src'};
      | def.LibPaths = {'C:\\prescandev\\vislibrary_build\lib'};
      | def.SampleTime = 'parameterized';
      | def.Options.language = 'C';
      mask Help: <p>This block was generated automatically by the Legacy Code Tool. For detailed help on this tool, call<a href="matlab:legacy_code('help')"> legacy_code('help')</a>.</p>
      mask Callback ShowSpec:
      | if strcmp(get_param(gcbh, 'ShowSpec'), 'on')
      |   set_param(gcbh, 'MaskDisplay', sprintf('fprintf(''%s'');', get_param(gcbh, 'SFunctionSpec')));
      | else
      |   set_param(gcbh, 'MaskDisplay', sprintf('fprintf(''%s'');', get_param(gcbh, 'FunctionName')));
      | end
      mask Display: fprintf('void prescan_synchronizer_outputFcn(void ** work1, PRESCAN_SYNCHRONIZEDATA y1[1])');
  wires:
  Bus Selector1/1 -> Stop Simulation/1  "<FederateStopped>"
  sfun_Synchronizer/1 -> Bus Selector1/1

== system Experiment_0310yice_cs/BMW_X5_SUV_1/Dynamics_Empty ==
  note: For state mode 'Dynamic' positions
      | are not taken into account, as they
      | are computed by integrating velocity.
      | Click annotation for Help.
  Ground_{1..9} (9 alike) : Ground
  MuxState : Subsystem  Tag=mux/State  mask(Empty Dynamics State Block){positioningmode=on, TimeStep=5/100}
      mask prompts: positioningmode "Positioning Mode"; TimeStep "Auto Assigned: Time Step [s]"
      mask help:
      | Build the state of an actor based on user input.
      | The user can either use positioning mode or dynamics mode.
      | - When using positioning mode the position and orientation of the actor are set directly based on the input. Expected input is relative to the initial position and orientation of the actor. It's also possible to specify the velocity of the actor, though this input isn't used, only passed on.
      | - When using dynamics mode the position input is ignored. Expected input is velocity and orientation. The velocity is relative the current orientation of the actor, while orientation is relative to its initial orientation. The position of the actor is calculated based on the velocity and orientation given.
      settings: DeleteFcn=PreScanBlockDeleteFcn;
  State : Outport  Tag=outport/StateOutport  SampleTime=5/100
  wires:
  MuxState/1(state) -> State/1
  Ground_1/1 -> MuxState/1(x [m])
  Ground_2/1 -> MuxState/2(y [m])
  Ground_3/1 -> MuxState/3(z [m])
  Ground_4/1 -> MuxState/4(dx [m/s])
  Ground_5/1 -> MuxState/5(dy [m/s])
  Ground_6/1 -> MuxState/6(dz [m/s])
  Ground_7/1 -> MuxState/7(R [rad])
  Ground_8/1 -> MuxState/8(P [rad])
  Ground_9/1 -> MuxState/9(Y [rad])

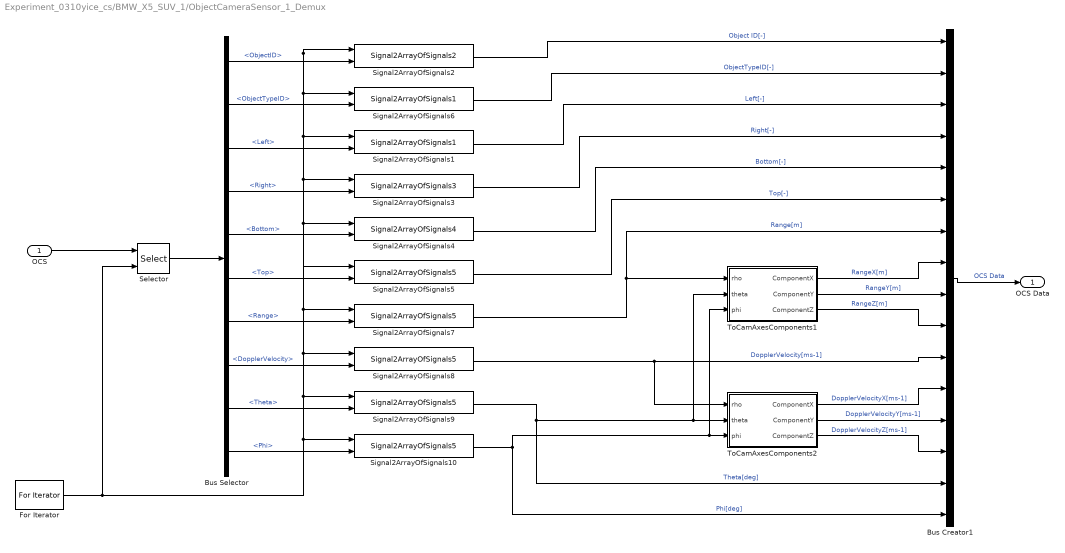
== system Experiment_0310yice_cs/BMW_X5_SUV_1/ObjectCameraSensor_1_Demux ==
  OCS : Inport
  Bus Creator1 : BusCreator  Inputs=16
  Bus Selector : BusSelector  OutputSignals=DATA.ObjectID,DATA.ObjectTypeID,DATA.Left,DATA.Right,DATA.Bottom,DATA.Top,DATA.Range,DATA.DopplerVelocity,DATA.Theta,DATA.Phi
  For Iterator : ForIterator  ResetStates=reset  IterationLimit=detectableObjects
  Selector : Selector  InputPortWidth=detectableObjects  IndexOptions=Index vector (port)  Indices=[1 3]  OutputSizes=1
  Signal2ArrayOfSignals1 : PreScanSimulinkLibrary/DemuxBRS/Signal2ArrayOfSignals1  VECTORLENGTH=detectableObjects
  Signal2ArrayOfSignals{5,7..10} (5 alike) : PreScanSimulinkLibrary/DemuxBRS/Signal2ArrayOfSignals5  VECTORLENGTH=detectableObjects
  Signal2ArrayOfSignals2 : PreScanSimulinkLibrary/DemuxBRS/Signal2ArrayOfSignals2  VECTORLENGTH=detectableObjects
  Signal2ArrayOfSignals3 : PreScanSimulinkLibrary/DemuxBRS/Signal2ArrayOfSignals3  VECTORLENGTH=detectableObjects
  Signal2ArrayOfSignals4 : PreScanSimulinkLibrary/DemuxBRS/Signal2ArrayOfSignals4  VECTORLENGTH=detectableObjects
  Signal2ArrayOfSignals6 : PreScanSimulinkLibrary/DemuxBRS/Signal2ArrayOfSignals1  VECTORLENGTH=detectableObjects
  ToCamAxesComponents1 : Subsystem
  ToCamAxesComponents2 : Subsystem
  OCS Data : Outport
  wires:
  OCS/1 -> Selector/1
  For Iterator/1 -> Selector/2, Signal2ArrayOfSignals2/1, Signal2ArrayOfSignals1/1, Signal2ArrayOfSignals3/1, Signal2ArrayOfSignals5/1, Signal2ArrayOfSignals4/1, Signal2ArrayOfSignals6/1, Signal2ArrayOfSignals7/1, Signal2ArrayOfSignals8/1, Signal2ArrayOfSignals9/1, Signal2ArrayOfSignals10/1
  Selector/1 -> Bus Selector/1
  Bus Selector/1 -> Signal2ArrayOfSignals2/2  "<ObjectID>"
  Bus Selector/3 -> Signal2ArrayOfSignals1/2  "<Left>"
  Bus Selector/4 -> Signal2ArrayOfSignals3/2  "<Right>"
  Bus Selector/5 -> Signal2ArrayOfSignals4/2  "<Bottom>"
  Bus Selector/6 -> Signal2ArrayOfSignals5/2  "<Top>"
  Signal2ArrayOfSignals2/1 -> Bus Creator1/1  "Object ID[-]"
  Signal2ArrayOfSignals1/1 -> Bus Creator1/3  "Left[-]"
  Signal2ArrayOfSignals6/1 -> Bus Creator1/2  "ObjectTypeID[-]"
  Signal2ArrayOfSignals3/1 -> Bus Creator1/4  "Right[-]"
  Bus Creator1/1 -> OCS Data/1  "OCS Data"
  Signal2ArrayOfSignals7/1 -> ToCamAxesComponents1/1(rho), Bus Creator1/7  "Range[m]"
  ToCamAxesComponents1/1(ComponentX) -> Bus Creator1/8  "RangeX[m]"
  ToCamAxesComponents1/2(ComponentY) -> Bus Creator1/9  "RangeY[m]"
  ToCamAxesComponents1/3(ComponentZ) -> Bus Creator1/10  "RangeZ[m]"
  ToCamAxesComponents2/1(ComponentX) -> Bus Creator1/12  "DopplerVelocityX[ms-1]"
  ToCamAxesComponents2/2(ComponentY) -> Bus Creator1/13  "DopplerVelocityY[ms-1]"
  ToCamAxesComponents2/3(ComponentZ) -> Bus Creator1/14  "DopplerVelocityZ[ms-1]"
  Signal2ArrayOfSignals9/1 -> Bus Creator1/15, ToCamAxesComponents2/2(theta), ToCamAxesComponents1/2(theta)  "Theta[deg]"
  Signal2ArrayOfSignals10/1 -> Bus Creator1/16, ToCamAxesComponents2/3(phi), ToCamAxesComponents1/3(phi)  "Phi[deg]"
  Bus Selector/2 -> Signal2ArrayOfSignals6/2  "<ObjectTypeID>"
  Bus Selector/7 -> Signal2ArrayOfSignals7/2  "<Range>"
  Bus Selector/8 -> Signal2ArrayOfSignals8/2  "<DopplerVelocity>"
  Bus Selector/9 -> Signal2ArrayOfSignals9/2  "<Theta>"
  Bus Selector/10 -> Signal2ArrayOfSignals10/2  "<Phi>"
  Signal2ArrayOfSignals8/1 -> ToCamAxesComponents2/1(rho), Bus Creator1/11  "DopplerVelocity[ms-1]"
  Signal2ArrayOfSignals4/1 -> Bus Creator1/5  "Bottom[-]"
  Signal2ArrayOfSignals5/1 -> Bus Creator1/6  "Top[-]"

== system Experiment_0310yice_cs/BMW_X5_SUV_1/ObjectCameraSensor_1_Image_Demux ==
  In1 : Inport
  Selector : Selector  NumberOfDimensions=2  InputPortWidth=3  IndexOptions=Index vector (dialog),Index vector (dialog)  Indices=-1,1:hres  OutputSizes=1,1
  Selector1 : Selector  NumberOfDimensions=2  InputPortWidth=3  IndexOptions=Index vector (dialog),Index vector (dialog)  Indices=-1,hres+1:hres*2  OutputSizes=1,1
  Selector2 : Selector  NumberOfDimensions=2  InputPortWidth=3  IndexOptions=Index vector (dialog),Index vector (dialog)  Indices=-1,hres*2+1:hres*3  OutputSizes=1,1
  R : Outport
  G : Outport  Port=2
  B : Outport  Port=3
  wires:
  In1/1 -> Selector1/1, Selector/1, Selector2/1
  Selector/1 -> R/1
  Selector1/1 -> G/1
  Selector2/1 -> B/1

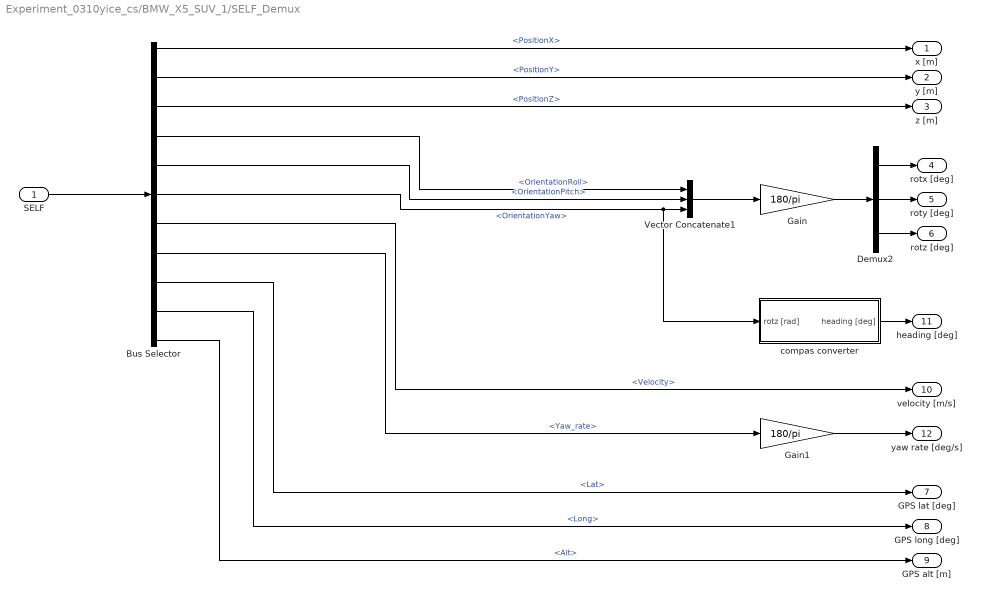
== system Experiment_0310yice_cs/BMW_X5_SUV_1/SELF_Demux ==
  SELF : Inport  OutDataTypeStr=Bus: PRESCAN_SELFSENSORDATA
  Bus Selector : BusSelector  OutputSignals=PositionX,PositionY,PositionZ,OrientationRoll,OrientationPitch,OrientationYaw,Velocity,Yaw_rate,Lat,Long,Alt
  Demux2 : Demux  Outputs=3
  Gain : Gain  Gain=180/pi
  Gain1 : Gain  Gain=180/pi
  Vector Concatenate1 : Concatenate  NumInputs=3
  compas converter : Subsystem
  x [m] : Outport
  y [m] : Outport  Port=2
  z [m] : Outport  Port=3
  rotx [deg] : Outport  Port=4
  roty [deg] : Outport  Port=5
  rotz [deg] : Outport  Port=6
  GPS lat [deg] : Outport  Port=7
  GPS long [deg] : Outport  Port=8
  GPS alt [m] : Outport  Port=9
  velocity [m/s] : Outport  Port=10
  heading [deg] : Outport  Port=11
  yaw rate [deg/s] : Outport  Port=12
  wires:
  Bus Selector/11 -> GPS alt [m]/1  "<Alt>"
  Bus Selector/10 -> GPS long [deg]/1  "<Long>"
  Bus Selector/9 -> GPS lat [deg]/1  "<Lat>"
  Bus Selector/8 -> Gain1/1  "<Yaw_rate>"
  Bus Selector/7 -> velocity [m/s]/1  "<Velocity>"
  Bus Selector/6 -> compas converter/1(rotz [rad]), Vector Concatenate1/3  "<OrientationYaw>"
  Bus Selector/5 -> Vector Concatenate1/2  "<OrientationPitch>"
  Bus Selector/4 -> Vector Concatenate1/1  "<OrientationRoll>"
  Vector Concatenate1/1 -> Gain/1
  Bus Selector/3 -> z [m]/1  "<PositionZ>"
  Bus Selector/2 -> y [m]/1  "<PositionY>"
  Bus Selector/1 -> x [m]/1  "<PositionX>"
  SELF/1 -> Bus Selector/1
  Gain/1 -> Demux2/1
  Demux2/1 -> rotx [deg]/1
  Demux2/2 -> roty [deg]/1
  Demux2/3 -> rotz [deg]/1
  compas converter/1(heading [deg]) -> heading [deg]/1
  Gain1/1 -> yaw rate [deg/s]/1

== system Experiment_0310yice_cs/BMW_X5_SUV_1/STATE_BMW_X5_SUV_1 ==
  State : Inport  SampleTime=TimeStep
  Bus Creator : BusCreator  Inputs=15  OutDataTypeStr=Bus: PRESCAN_STATEACTUATORDATA  NonVirtualBus=on
  Demux : Demux  Outputs=15
  iniBODYAngles wrtVEH [rad] : Constant  Value=[Roll0 Pitch0 0]  SampleTime=TimeStep
  iniVEHAngles wrtGLOB [rad] : Constant  Value=[0 0 Yaw0]  SampleTime=TimeStep
  iniVEHposition wrtGLOB [m] : Constant  Value=[x0 y0 z0]  SampleTime=TimeStep
  state2FullState : PreScanSimulinkLibrary/state2FullState  SystemSampleTime=-1
  StateBus : Outport  OutDataTypeStr=Bus: PRESCAN_STATEACTUATORDATA
  wires:
  Bus Creator/1 -> StateBus/1
  State/1 -> state2FullState/1
  state2FullState/1 -> Demux/1
  iniVEHposition wrtGLOB [m]/1 -> state2FullState/2
  iniBODYAngles wrtVEH [rad]/1 -> state2FullState/3
  iniVEHAngles wrtGLOB [rad]/1 -> state2FullState/4
  Demux/1 -> Bus Creator/1  "PositionX"
  Demux/2 -> Bus Creator/2  "PositionY"
  Demux/3 -> Bus Creator/3  "PositionZ"
  Demux/4 -> Bus Creator/4  "VelocityX"
  Demux/5 -> Bus Creator/5  "VelocityY"
  Demux/6 -> Bus Creator/6  "VelocityZ"
  Demux/7 -> Bus Creator/7  "AccelerationX"
  Demux/8 -> Bus Creator/8  "AccelerationY"
  Demux/9 -> Bus Creator/9  "AccelerationZ"
  Demux/10 -> Bus Creator/10  "OrientationRoll"
  Demux/11 -> Bus Creator/11  "OrientationPitch"
  Demux/12 -> Bus Creator/12  "OrientationYaw"
  Demux/13 -> Bus Creator/13  "AngularVelocityRoll"
  Demux/14 -> Bus Creator/14  "AngularVelocityPitch"
  Demux/15 -> Bus Creator/15  "AngularVelocityYaw"

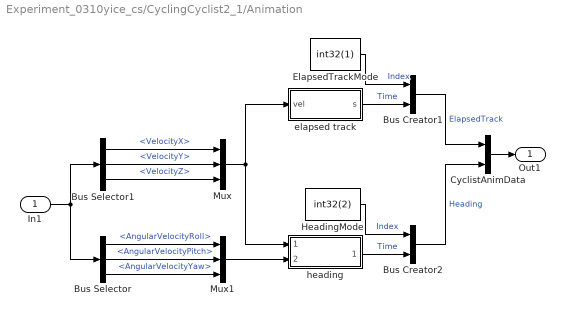
== system Experiment_0310yice_cs/CyclingCyclist2_1/Animation ==
  In1 : Inport  OutDataTypeStr=Bus: PRESCAN_STATEACTUATORDATA
  Bus Creator1 : BusCreator  Inputs=2  OutDataTypeStr=Bus: PRESCAN_ANIMACTUATORDATA  NonVirtualBus=on
  Bus Creator2 : BusCreator  Inputs=2  OutDataTypeStr=Bus: PRESCAN_ANIMACTUATORDATA  NonVirtualBus=on
  Bus Selector : BusSelector  OutputSignals=AngularVelocityRoll,AngularVelocityPitch,AngularVelocityYaw
  Bus Selector1 : BusSelector  OutputSignals=VelocityX,VelocityY,VelocityZ
  CyclistAnimData : Concatenate
  ElapsedTrackMode : Constant  Value=int32(1)
  HeadingMode : Constant  Value=int32(2)
  Mux : Mux  Inputs=3
  Mux1 : Mux  Inputs=3
  elapsed track : Subsystem
  heading : Subsystem
  Out1 : Outport  OutDataTypeStr=Bus: PRESCAN_ANIMACTUATORDATA
  wires:
  In1/1 -> Bus Selector/1, Bus Selector1/1
  CyclistAnimData/1 -> Out1/1
  Bus Selector1/1 -> Mux/1  "<VelocityX>"
  Bus Selector1/2 -> Mux/2  "<VelocityY>"
  Bus Selector1/3 -> Mux/3  "<VelocityZ>"
  Bus Selector/1 -> Mux1/1  "<AngularVelocityRoll>"
  Bus Selector/2 -> Mux1/2  "<AngularVelocityPitch>"
  Bus Selector/3 -> Mux1/3  "<AngularVelocityYaw>"
  Mux/1 -> elapsed track/1(vel), heading/1(velocity)
  Mux1/1 -> heading/2(velRPY)
  heading/1(heading) -> Bus Creator2/2  "Time"
  Bus Creator2/1 -> CyclistAnimData/2  "Heading"
  Bus Creator1/1 -> CyclistAnimData/1  "ElapsedTrack"
  HeadingMode/1 -> Bus Creator2/1  "Index"
  elapsed track/1(s) -> Bus Creator1/2  "Time"
  ElapsedTrackMode/1 -> Bus Creator1/1  "Index"

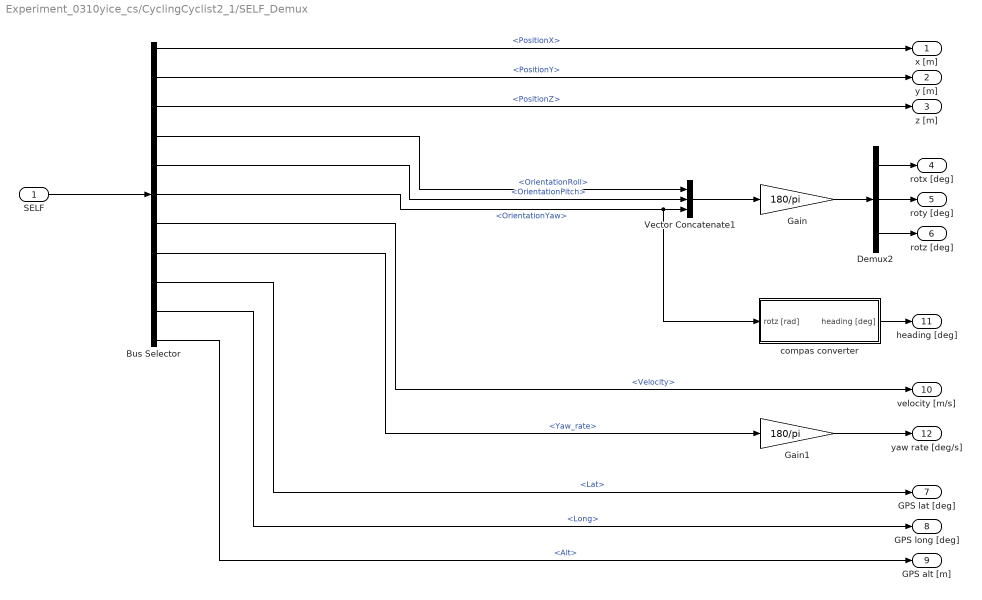
== system Experiment_0310yice_cs/CyclingCyclist2_1/SELF_Demux ==
  SELF : Inport  OutDataTypeStr=Bus: PRESCAN_SELFSENSORDATA
  Bus Selector : BusSelector  OutputSignals=PositionX,PositionY,PositionZ,OrientationRoll,OrientationPitch,OrientationYaw,Velocity,Yaw_rate,Lat,Long,Alt
  Demux2 : Demux  Outputs=3
  Gain : Gain  Gain=180/pi
  Gain1 : Gain  Gain=180/pi
  Vector Concatenate1 : Concatenate  NumInputs=3
  compas converter : Subsystem
  x [m] : Outport
  y [m] : Outport  Port=2
  z [m] : Outport  Port=3
  rotx [deg] : Outport  Port=4
  roty [deg] : Outport  Port=5
  rotz [deg] : Outport  Port=6
  GPS lat [deg] : Outport  Port=7
  GPS long [deg] : Outport  Port=8
  GPS alt [m] : Outport  Port=9
  velocity [m/s] : Outport  Port=10
  heading [deg] : Outport  Port=11
  yaw rate [deg/s] : Outport  Port=12
  wires:
  Bus Selector/11 -> GPS alt [m]/1  "<Alt>"
  Bus Selector/10 -> GPS long [deg]/1  "<Long>"
  Bus Selector/9 -> GPS lat [deg]/1  "<Lat>"
  Bus Selector/8 -> Gain1/1  "<Yaw_rate>"
  Bus Selector/7 -> velocity [m/s]/1  "<Velocity>"
  Bus Selector/6 -> compas converter/1(rotz [rad]), Vector Concatenate1/3  "<OrientationYaw>"
  Bus Selector/5 -> Vector Concatenate1/2  "<OrientationPitch>"
  Bus Selector/4 -> Vector Concatenate1/1  "<OrientationRoll>"
  Vector Concatenate1/1 -> Gain/1
  Bus Selector/3 -> z [m]/1  "<PositionZ>"
  Bus Selector/2 -> y [m]/1  "<PositionY>"
  Bus Selector/1 -> x [m]/1  "<PositionX>"
  SELF/1 -> Bus Selector/1
  Gain/1 -> Demux2/1
  Demux2/1 -> rotx [deg]/1
  Demux2/2 -> roty [deg]/1
  Demux2/3 -> rotz [deg]/1
  compas converter/1(heading [deg]) -> heading [deg]/1
  Gain1/1 -> yaw rate [deg/s]/1
